simulink model "elbow_manipulator_model"  (R2017a)
settings: Solver=ode45  StartTime=0.0  StopTime=T  RelTol=2.8421709430404007E-14  AbsTol=2.8421709430404007E-14
values from neighbouring files (symbols this model uses):
  fs_1 = 0.1    [Two_DOF_Manipulator.m]
  fs_2 = 0.1    [Two_DOF_Manipulator.m]
  g = 9.8    [Two_DOF_Manipulator.m]
  L_1 = 1    [Two_DOF_Manipulator.m]
  L_2 = 0.5    [Two_DOF_Manipulator.m]
  m_1 = 1    [Two_DOF_Manipulator.m]
  m_2 = 2    [Two_DOF_Manipulator.m]
  theta1_0 = beta    (= 0)    [Two_DOF_Manipulator.m]
  theta2_0 = alpha    (= -2.35619449019)    [Two_DOF_Manipulator.m]
  theta_1_max = pi    (= 3.14159265359)    [Two_DOF_Manipulator.m]
  theta_1_min = 0    [Two_DOF_Manipulator.m]
  theta_2_max = 3*pi/4    (= 2.35619449019)    [Two_DOF_Manipulator.m]
  theta_2_min = -3*pi/4    (= -2.35619449019)    [Two_DOF_Manipulator.m]
settings Model: Creator=cc16g15  LastModifiedBy=cchoc
settings SolverCC: MaxConsecutiveMinStep=1000  ZeroCrossControl=DisableAll  ZeroCrossAlgorithm=Adaptive

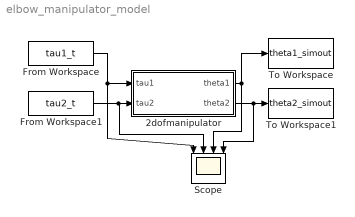
== system elbow_manipulator_model ==
  2dofmanipulator : Subsystem
  From Workspace : FromWorkspace  VariableName=tau1_t  OutDataTypeStr=double  OutputAfterFinalValue=Setting to zero
  From Workspace1 : FromWorkspace  VariableName=tau2_t  OutDataTypeStr=double  OutputAfterFinalValue=Setting to zero
  Scope : Scope  NumInputPorts=4
  To Workspace : ToWorkspace  VariableName=theta1_simout  SaveFormat=Timeseries  SampleTime=-1
  To Workspace1 : ToWorkspace  VariableName=theta2_simout  SaveFormat=Timeseries  SampleTime=-1
  wires:
  From Workspace/1 -> 2dofmanipulator/1(tau1), Scope/1
  From Workspace1/1 -> Scope/2, 2dofmanipulator/2(tau2)
  2dofmanipulator/2(theta2) -> To Workspace1/1, Scope/4
  2dofmanipulator/1(theta1) -> To Workspace/1, Scope/3

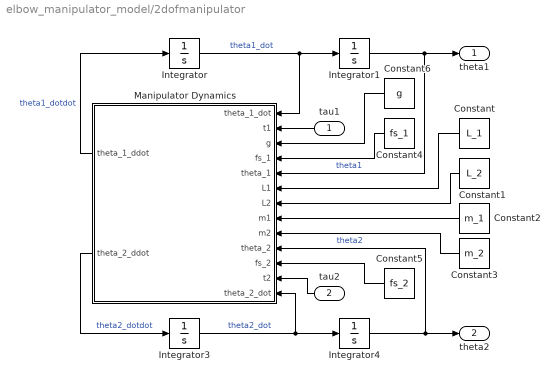
== system elbow_manipulator_model/2dofmanipulator ==
  tau1 : Inport
  tau2 : Inport  Port=2
  Constant : Constant  Value=L_1
  Constant1 : Constant  Value=L_2
  Constant2 : Constant  Value=m_1
  Constant3 : Constant  Value=m_2
  Constant4 : Constant  Value=fs_1
  Constant5 : Constant  Value=fs_2
  Constant6 : Constant  Value=g
  Integrator : Integrator  InitialCondition=0.000001  ZeroCross=off
  Integrator1 : Integrator  InitialCondition=theta1_0  LimitOutput=on  UpperSaturationLimit=theta_1_max  LowerSaturationLimit=theta_1_min  ZeroCross=off
  Integrator3 : Integrator  ZeroCross=off
  Integrator4 : Integrator  InitialCondition=theta2_0  LimitOutput=on  UpperSaturationLimit=theta_2_max  LowerSaturationLimit=theta_2_min  ZeroCross=off
  Manipulator Dynamics : MATLAB Function  TreatAsAtomicUnit=on
  theta1 : Outport
  theta2 : Outport  Port=2
  wires:
  Integrator1/1 -> theta1/1, Manipulator Dynamics/5(theta_1)  "theta1"
  Manipulator Dynamics/2(theta_2_ddot) -> Integrator3/1  "theta2_dotdot"
  Integrator/1 -> Manipulator Dynamics/1(theta_1_dot), Integrator1/1  "theta1_dot"
  Integrator3/1 -> Manipulator Dynamics/13(theta_2_dot), Integrator4/1  "theta2_dot"
  Manipulator Dynamics/1(theta_1_ddot) -> Integrator/1  "theta1_dotdot"
  Integrator4/1 -> Manipulator Dynamics/10(theta_2), theta2/1  "theta2"
  Constant3/1 -> Manipulator Dynamics/9(m2)
  Constant2/1 -> Manipulator Dynamics/8(m1)
  Constant1/1 -> Manipulator Dynamics/7(L2)
  Constant/1 -> Manipulator Dynamics/6(L1)
  tau1/1 -> Manipulator Dynamics/2(t1)
  tau2/1 -> Manipulator Dynamics/12(t2)
  Constant5/1 -> Manipulator Dynamics/11(fs_2)
  Constant4/1 -> Manipulator Dynamics/4(fs_1)
  Constant6/1 -> Manipulator Dynamics/3(g)

== matlab function elbow_manipulator_model/2dofmanipulator/Manipulator Dynamics ==
  data: theta_1_dot input; t1 input; g input; fs_1 input; theta_1 input; L1 input; L2 input; m1 input; m2 input; theta_1_ddot output; theta_2_ddot output; theta_2 input; fs_2 input; t2 input; theta_2_dot input
function [theta_1_ddot,theta_2_ddot] = fcn(theta_1_dot,t1,g, fs_1,theta_1,L1,L2,m1,m2,theta_2 ,fs_2,t2,theta_2_dot)

M = [m1*L1^2+m2*(L1^2+L2^2+2*L1*L2*cos(theta_2)) m2*(L2^2+L1*L2*cos(theta_2));...
    m2*(L2^2+L1*L2*cos(theta_2)) m2*L2^2]; 
C = [theta_2_dot*(-2*m2*L1*L2*sin(theta_2)) theta_2_dot*(-m2*L1*L2*sin(theta_2));...
    theta_1_dot*(m2*L1*L2*sin(theta_2)) 0];
G = [-g*L1*(m1+m2)*cos(theta_1)-m2*g*L2*cos(theta_1+theta_2); -m2*g*L2*cos(theta_1+theta_2)];

theta_ddot = M\([t1;t2]-C*[theta_1_dot;theta_2_dot]...
    -[fs_1*sign(theta_1_dot); fs_2*sign(theta_2_dot)]-G);

theta_1_ddot = theta_ddot(1,1);
theta_2_ddot = theta_ddot(2,1);
end
